simulink model "W05_G_tuning"  (R2024b)
settings: Solver=ode4  StartTime=0  StopTime=T_final  FixedStep=h  RelTol=1e-3
InitFcn:
  | if base_var('pace', 0) > 0, set_param(bdroot, 'EnablePacing', 'on', 'PacingRate', '1'); else, set_param(bdroot, 'EnablePacing', 'off'); end
StopFcn:
  | W05_plot;
values from neighbouring files (symbols this model uses):
  animate = 1    [W05_0_setup.m]
  beta_c = pi/2    (= 1.57079632679)    [W05_0_setup.m]
  Delta = 5    [W05_0_setup.m]
  k_neg = cfg.k_neg    [W05_0_setup.m]
  k_pos = cfg.k_pos    [W05_0_setup.m]
  kappa = 0.3    [W05_0_setup.m]    (also in W05_G_tuning_by_hand.m = 0 이면 LOS 와 같다 / 0 is LOS)
  Kd = 100    [W05_0_setup.m]
  Kp = 300    [W05_0_setup.m]
  mp = 25    [W05_0_setup.m]
  n_max = cfg.n_max    [W05_0_setup.m]
  N_max = N_lim(X_ff)    [W05_0_setup.m]
  n_min = cfg.n_min    [W05_0_setup.m]
  R_switch = 3    [W05_0_setup.m]
  rp = [0.05 0 -0.35]'    [W05_0_setup.m]
  V_c = 0    [W05_0_setup.m]
  WP_E = [0  0 60 60 120]'    [W05_0_setup.m]    (also in W05_plot.m = evalin('base','WP_E'))
  WP_N = [0 60 60  0  60]'    [W05_0_setup.m]    (also in W05_plot.m = evalin('base','WP_N'))
  x0 = zeros(12,1);  x0(8) = E0    [W05_0_setup.m]
  X_ff = 60    [W05_0_setup.m]
  y_pont = cfg.y_pont    [W05_0_setup.m]
settings Model: Creator=admin  LastModifiedBy=admin
settings DataIOCC: ReturnWorkspaceOutputs=off

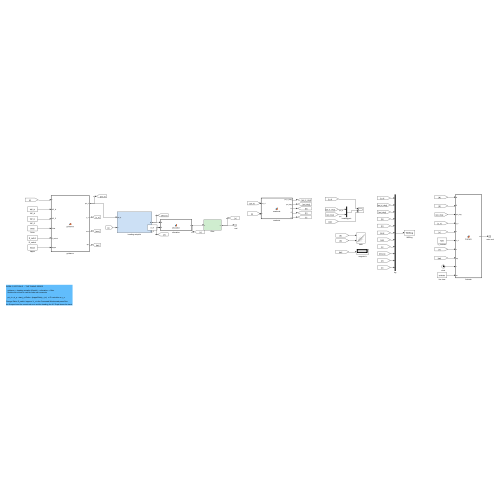
[thumbnail: Simulink's stored preview of the top-level diagram]
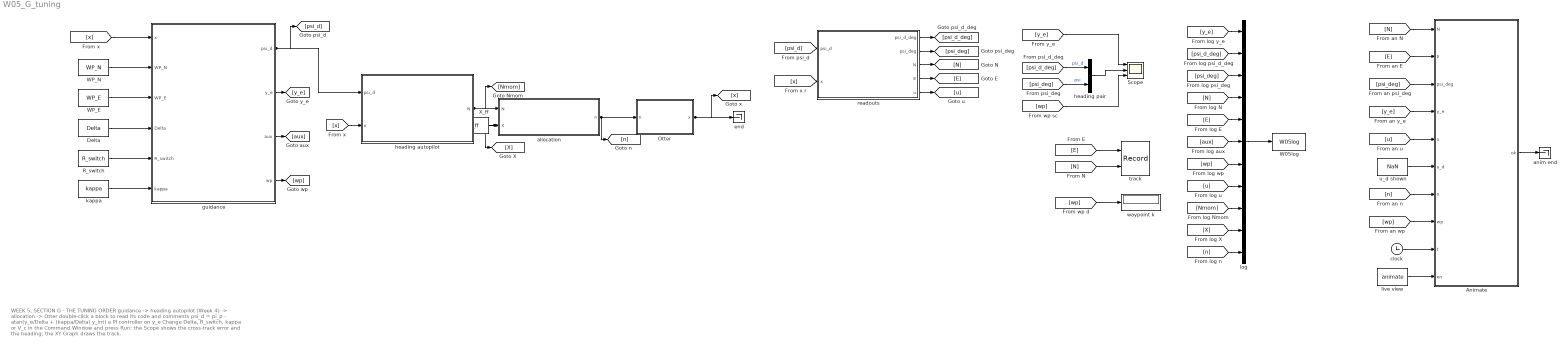
== system W05_G_tuning ==
  note: WEEK 5, SECTION G  -  THE TUNING ORDER
      |
      |    guidance -> heading autopilot (Week 4) -> allocation -> Otter
      |    double-click a block to read its code and comments
      |
      |    psi_d = pi_p - atan(y_e/Delta + (kappa/Delta) y_int)   a PI controller on y_e
      |
      | Change Delta, R_switch, kappa or V_c in the Command Window and press Run:
      | the Scope shows the cross-track error and the heading; the XY Graph draws the track.
  Animate : MATLAB Function  TreatAsAtomicUnit=on
  Delta : Constant  Value=Delta
  Otter : Subsystem
  R_switch : Constant  Value=R_switch
  Scope : Scope  NumInputPorts=3
  W05log : ToWorkspace  VariableName=W05log  SaveFormat=Structure With Time  SampleTime=-1
  WP_E : Constant  Value=WP_E
  WP_N : Constant  Value=WP_N
  X_ff : Constant  Value=X_ff
  allocation : MATLAB Function  TreatAsAtomicUnit=on
  anim end : Terminator
  clock : Clock
  end : Terminator
  guidance : MATLAB Function  TreatAsAtomicUnit=on
  heading autopilot : Subsystem
  heading pair : Mux  Inputs=2
  kappa : Constant  Value=kappa
  live view : Constant  Value=animate
  log : Mux  Inputs=11
  readouts : MATLAB Function  TreatAsAtomicUnit=on
  track : Record  FileSettingsInternal="{\"entries\":[{\"content\":{\"excelSettings\":{\"content\":{},\"type\":\"Streamout.ExcelSettings\"}},\"type\":\"Streamout.FileSettingStorage\",\"uuid\":\"\"}],\"packageUris\":[\"http:\\/\\/schema.mathworks.com\\/mf0\\/streamout_blocks\\/R2020a\"],\"version\":\"1.0\"}"  Layout=[1 1]  SignalsInternal="{\"entries\":[{\"content\":{\"signals\":[{\"content\":{\"blockPath\":[],\"dimensions\":[1],\"domain\":\"\",\"lineColor\":\"#a2142f\",\"plots\":[ 1 ],\"port\":1,\"signalID\":1,\"signalName\":\"XY Graph:1\"},\"type\":\"RecordBlkView.Signal\",\"uuid\":\"\"},{\"content\":{\"blockPath\":[],\"dimensions\":[1],\"domain\":\"\",\"lineColor\":\"#139fff\",\"plots\":[ 1 ],\"port\":2,\"signalID\":2,\"signalName\":\"XY Graph:2\"},\"type\":\"RecordBlkView.Signal\",\"uuid\":\"\"}]},\"type\":\"RecordBlkView.InputSignals\",\"uuid\":\"\"}],\"packageUris\":[\"http:\\/\\/schema.mathworks.com\\/mf0\\/streamout_blocks\\/R2020a\"],\"version\":\"1.0\"}"  VisualizationBindings="{\"xyplotplugin\":{\"info\":[{\"series\":[{\"bindingParametersList\":[{\"parameter\":\"X-Axis\",\"signalID\":1,\"signalName\":\"XY Graph:1\"},{\"parameter\":\"Y-Axis\",\"signalID\":2,\"signalName\":\"XY Graph:2\"}],\"seriesID\":0}],\"subplotID\":1}]}}"  CompatibilityTag=XY
  u_d shown : Constant  Value=NaN
  waypoint k : Display
  wires:
  [x] -> guidance/1(x)
  WP_N/1 -> guidance/2(WP_N)
  WP_E/1 -> guidance/3(WP_E)
  Delta/1 -> guidance/4(Delta)
  R_switch/1 -> guidance/5(R_switch)
  kappa/1 -> guidance/6(kappa)
  guidance/1(psi_d) -> heading autopilot/1(psi_d), [psi_d]
  [x] -> heading autopilot/2(x)
  guidance/2(y_e) -> [y_e]
  guidance/3(aux) -> [aux]
  guidance/4(wp) -> [wp]
  heading autopilot/1(N) -> allocation/1(N), [Nmom]
  X_ff/1 -> allocation/2(X), [X]
  allocation/1(n) -> Otter/1(n), [n]
  Otter/1(x) -> [x], end/1
  [psi_d] -> readouts/1(psi_d)
  [x] -> readouts/2(x)
  readouts/1(psi_d_deg) -> [psi_d_deg]
  readouts/2(psi_deg) -> [psi_deg]
  readouts/3(N) -> [N]
  readouts/4(E) -> [E]
  readouts/5(u) -> [u]
  [y_e] -> Scope/1
  [psi_d_deg] -> heading pair/1  "psi_d"
  [psi_deg] -> heading pair/2  "psi"
  heading pair/1 -> Scope/2
  [wp] -> Scope/3
  [E] -> track/1
  [N] -> track/2
  [wp] -> waypoint k/1
  [N] -> Animate/1(N)
  [E] -> Animate/2(E)
  [psi_deg] -> Animate/3(psi_deg)
  [y_e] -> Animate/4(y_e)
  [u] -> Animate/5(u)
  u_d shown/1 -> Animate/6(u_d)
  [n] -> Animate/7(n)
  [wp] -> Animate/8(wp)
  clock/1 -> Animate/9(t)
  live view/1 -> Animate/10(en)
  Animate/1(ok) -> anim end/1
  [y_e] -> log/1
  [psi_d_deg] -> log/2
  [psi_deg] -> log/3
  [N] -> log/4
  [E] -> log/5
  [aux] -> log/6
  [wp] -> log/7
  [u] -> log/8
  [Nmom] -> log/9
  [X] -> log/10
  [n] -> log/11
  log/1 -> W05log/1

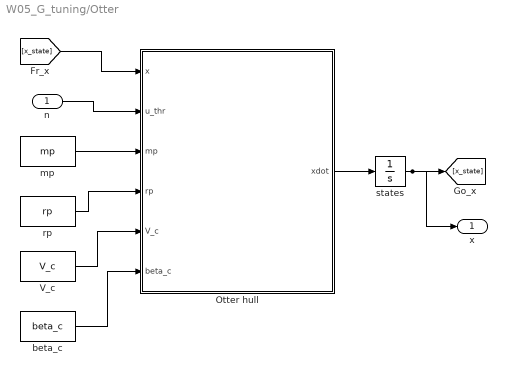
== system W05_G_tuning/Otter ==
  n : Inport
  Otter hull : MATLAB Function  TreatAsAtomicUnit=on
  V_c : Constant  Value=V_c
  beta_c : Constant  Value=beta_c
  mp : Constant  Value=mp
  rp : Constant  Value=rp
  states : Integrator  InitialCondition=x0
  x : Outport
  wires:
  [x_state] -> Otter hull/1(x)
  states/1 -> [x_state], x/1
  n/1 -> Otter hull/2(u_thr)
  mp/1 -> Otter hull/3(mp)
  rp/1 -> Otter hull/4(rp)
  Otter hull/1(xdot) -> states/1
  V_c/1 -> Otter hull/5(V_c)
  beta_c/1 -> Otter hull/6(beta_c)

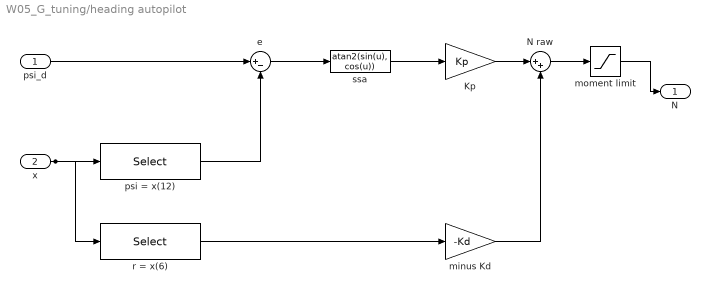
== system W05_G_tuning/heading autopilot ==
  psi_d : Inport
  x : Inport  Port=2
  Kp : Gain  Gain=Kp
  N raw : Sum  Inputs=|++
  e : Sum  Inputs=|+-
  minus Kd : Gain  Gain=-Kd
  moment limit : Saturate  UpperLimit=N_max  LowerLimit=-N_max
  psi = x(12) : Selector  InputPortWidth=12  IndexOptions=Index vector (dialog)  Indices=12  OutputSizes=1
  r = x(6) : Selector  InputPortWidth=12  IndexOptions=Index vector (dialog)  Indices=6  OutputSizes=1
  ssa : Fcn  Expr=atan2(sin(u), cos(u))
  N : Outport
  wires:
  x/1 -> psi = x(12)/1, r = x(6)/1
  psi_d/1 -> e/1
  psi = x(12)/1 -> e/2
  e/1 -> ssa/1
  ssa/1 -> Kp/1
  r = x(6)/1 -> minus Kd/1
  Kp/1 -> N raw/1
  minus Kd/1 -> N raw/2
  N raw/1 -> moment limit/1
  moment limit/1 -> N/1

== matlab function W05_G_tuning/allocation ==
  data: N input; n output double size=[2 1]; X input; y_pont parameter; k_pos parameter; k_neg parameter; n_max parameter; n_min parameter
function n = allocation(N, X, y_pont, k_pos, k_neg, n_max, n_min)
%#codegen
%ALLOCATION  전진력 X 와 요 모멘트 N 을 두 축의 회전수 n = [n_L; n_R] 로.
%            The surge force X and the yaw moment N to the two shaft speeds.
%  X 는 상수 X_ff 다 - 캔버스의 Constant 블록이 넣어 준다.
%  X is the constant X_ff, put in by a Constant block on the canvas.

% 1) 두 힘을 두 추력으로. 배치행렬 B 를 세우고 **풀면** 된다 - 손으로 푼
%    T = X/2 +- N/(2 y_pont) 와 같은 것이고, 이 쪽이 5-7 절의 유도와 같은
%    모양이다. MSS 데모도 이렇게 한다: demoOtterUSVPathFollowingHeadingControl
%    의 Allocation 안에 Constant [1 1; 0.395 -0.395] 와 행렬 나눗셈이 있다.
%    B is square and nonsingular here, so the two forces are shared by solving
%    rather than by two hand-written expressions. The MSS demonstration model
%    does the same: its Allocation holds the constant [1 1; 0.395 -0.395] and
%    a matrix division.
B = [1        1;              % 전진력  X = T_L + T_R        / surge force
     y_pont  -y_pont];        % 요 모멘트 N = y_pont(T_L-T_R) / yaw moment
T = B \ [X; N];               % 좌현, 우현 / port, starboard

% 2) 프로펠러 곡선 T = k n|n| 을 n 에 대해 푼다 (앞 k_pos, 뒤 k_neg).
%    Solve the propeller curve T = k n|n| for n (k_pos ahead, k_neg astern).
n = zeros(2,1);
for i = 1:2
    if T(i) >= 0
        n(i) =  sqrt( T(i) / k_pos);
    else
        n(i) = -sqrt(-T(i) / k_neg);
    end
end

% 3) 프로펠러가 낼 수 있는 범위로 자른다. **otter.m 이 안에서 이미 자르기 때문에**
%    (MSS otter.m 167-170 행) 여기서 자르지 않으면 로그에 적히는 n 이 플랜트가
%    실제로 받은 n 과 달라진다 - 기록은 플랜트가 받은 것이어야 한다.
%    Clamp to what the propellers can do. otter.m clamps internally (lines
%    167-170), so without this the logged n would not be the n the plant got,
%    and a log must record what the plant received.
n(1) = min(max(n(1), n_min), n_max);
n(2) = min(max(n(2), n_min), n_max);
end

== matlab function W05_G_tuning/guidance ==
  settings: updateMethod=DISCRETE  sampleTime=h
  data: x input; psi_d output double size=[1 1]; WP_N input; WP_E input; Delta input; R_switch input; kappa input; y_e output; aux output; wp output; h parameter
function [psi_d, y_e, aux, wp] = guidance(x, WP_N, WP_E, Delta, R_switch, kappa, h)
%#codegen
%GUIDANCE  웨이포인트 목록과 배의 위치에서 명령 선수각 psi_d 를 만든다.
%          Make the commanded heading psi_d from the waypoint list and the position.
%
%   입력 x 는 Otter 의 12 상태 (위치 N = x(7), E = x(8)). 나머지는 작업공간 변수.
%   The input x is the Otter's 12 states (position N = x(7), E = x(8));
%   the rest are workspace variables (W05_0_setup).
%
%   출력 / outputs
%     psi_d  명령 선수각 [rad] -> 선수각 오토파일럿 / commanded heading -> the autopilot
%     y_e    횡방향 오차 [m], 경로 오른쪽이 + / cross-track error, right of the path +
%     aux    ILOS 의 적분 상태 (다른 법칙은 0) / the ILOS integral (0 for other laws)
%     wp     지금 따라가는 다리 번호 / the leg being followed

% 0) 기억하는 값: 지금 다리 k, 적분 y_int. 블록이 가지고 있다가 실행마다 처음으로 돌아간다.
%    Remembered values: the leg k and the integral y_int. The block owns them,
%    and they start afresh on every run.
persistent k y_int
if isempty(k), k = 1; y_int = 0; end
N = x(7);  E = x(8);
n = numel(WP_N);

% 1) 지금 다리: 웨이포인트 k 에서 k+1 로. 그 방향이 경로 각 pi_p 다.
%    The active leg runs from waypoint k to k+1; its direction is the path angle pi_p.
kn = min(k+1, n);
Nk = WP_N(k);   Ek = WP_E(k);
Nn = WP_N(kn);  En = WP_E(kn);
pi_p = atan2(En - Ek, Nn - Nk);

% 2) 배의 위치를 경로 좌표로 돌린다: x_e = 다리를 따라 간 거리, y_e = 다리에서 옆으로 벗어난 거리.
%    Rotate the position into path coordinates: x_e = distance along the leg,
%    y_e = distance off it, to the side.
dN = N - Nk;  dE = E - Ek;
x_e =  dN*cos(pi_p) + dE*sin(pi_p);
y_e = -dN*sin(pi_p) + dE*cos(pi_p);

% 3) 다리 끝까지 R_switch 보다 적게 남으면 다음 다리로 (MSS 와 같은 판정).
%    With less than R_switch left to the end of the leg, move to the next leg
%    (the same test as MSS).
d = sqrt((Nn - Nk)^2 + (En - Ek)^2);
if (d - x_e) < R_switch && k < n-1
    k = k + 1;
end
wp = k;
aux = y_int;

% 4) 법칙 ILOS: LOS 에 적분을 더한다 — 횡방향 오차에 대한 PI 제어기.
%        psi_d = pi_p - atan(y_e/Delta + (kappa/Delta) y_int)
%    조류가 배를 계속 밀면 LOS 는 오차를 남긴다 (P 가 남기는 오차와 같다). 적분이 그만큼을 맡는다.
%    The law ILOS: LOS plus an integral — a PI controller on the cross-track
%    error. A current that keeps pushing leaves an error with LOS alone (the
%    error P leaves); the integral takes it over.
psi_d = pi_p - atan(y_e/Delta + (kappa/Delta)*y_int);

% 5) 적분 갱신. 분모가 y_e 와 함께 커지므로 멀리 벗어나 있을 때는 거의 적분하지 않는다:
%    법칙 안에 들어 있는 안티와인드업이다 (Borhaug, Pavlov, Pettersen 2008).
%    Update the integral. The denominator grows with y_e, so it barely
%    integrates while far off the path: anti-windup built into the law.
y_int = y_int + h * Delta*y_e / (Delta^2 + (y_e + kappa*y_int)^2);
end

== matlab function W05_G_tuning/Otter/Otter hull ==
  data: x input; xdot output double size=[12 1]; u_thr input; mp input; rp input; V_c input; beta_c input
function xdot = otter_hull(x, u_thr, mp, rp, V_c, beta_c)
% Fossen's otter.m, called unchanged from Tools/MSS/VESSELS.
%
%   x       12 states, fed back from the integrator
%   u_thr   propeller shaft speeds [rad/s]
%
% otter.m is not written for code generation, so the call is extrinsic and
% xdot has to be pre-sized for Simulink to know the output width.
coder.extrinsic('otter');

xdot = zeros(12,1);
xdot = otter(x, u_thr, mp, rp, V_c, beta_c);
end

== matlab function W05_G_tuning/readouts ==
  data: psi_d input; psi_d_deg output double size=[1 1]; x input; psi_deg output; N output; E output; u output
function [psi_d_deg, psi_deg, N, E, u] = readouts(psi_d, x)
%#codegen
%READOUTS  Scope 와 XY Graph 에 보낼 값을 꺼낸다. 제어에는 쓰지 않는다.
%          Pick out what the Scope and the XY Graph show; not used for control.

% 1) 명령 선수각을 도로 / the commanded heading in degrees
psi_d_deg = psi_d * 180/pi;

% 2) 선수각은 x(12). 여러 번 돌면 360 도를 넘으므로 (-180, 180] 로 감아 psi_d 와 같은 범위로.
%    The heading is x(12); after turns it passes 360 deg, so it is wrapped into
%    (-180, 180], the range of psi_d.
psi_deg = atan2(sin(x(12)), cos(x(12))) * 180/pi;

% 3) 위치: 북 x(7), 동 x(8) / position: north x(7), east x(8)
N = x(7);  E = x(8);

% 4) 전진속도 x(1). 대부분의 모델에서는 X_ff 가 정한 값이 그대로 나오고,
%    §5-7 의 W05_H_speed_path 에서만 속도 루프가 이것을 붙든다.
%    Surge speed, state 1. In most models it is whatever X_ff produces; only in
%    W05_H_speed_path of §5-7 is it held by a controller.
u = x(1);
end

== matlab function W05_G_tuning/Animate ==
  data: N input; E input; psi_deg input; y_e input; u input; ok output double size=[1 1]; u_d input; n input; wp input; t input; en input
function ok = Animate(N, E, psi_deg, y_e, u, u_d, n, wp, t, en)
%#codegen
%ANIMATE  도는 동안의 실시간 화면 / the live view, while the model runs.
%
%  MATLAB Function 블록은 그림을 그릴 수 없다. 그래서 그리는 함수를 extrinsic 으로
%  선언한다 — Simulink 가 코드를 생성하지 않고 평범한 MATLAB 을 부른다.
%  A MATLAB Function block cannot plot, so the drawing function is declared
%  extrinsic: Simulink calls plain MATLAB instead of generating code for it.
%
%  en = animate (작업공간). 0 이면 이 블록은 아무것도 하지 않는다.
%  en is the workspace variable animate; at 0 this block does nothing.
coder.extrinsic('W05_animate');
ok = 1;
if en > 0.5
    W05_animate(N, E, psi_deg, y_e, u, u_d, n, wp, t);
end
end
